simulink model "LotkaVolterra"  (R2024b)
settings: Solver=VariableStepAuto  StartTime=0.0  StopTime=10.0  RelTol=1e-3
settings Model: Creator=hp  LastModifiedBy=hp
settings DataIOCC: ReturnWorkspaceOutputs=off

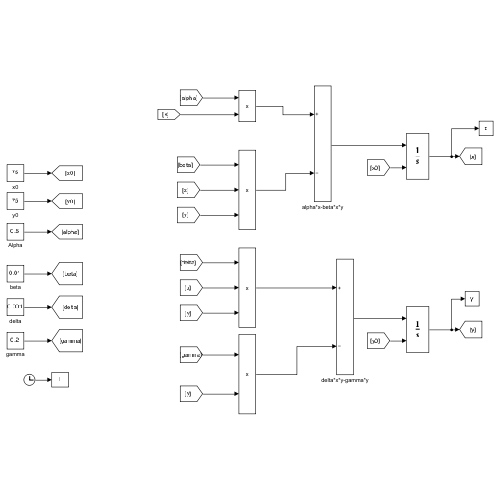
[thumbnail: Simulink's stored preview of the top-level diagram]
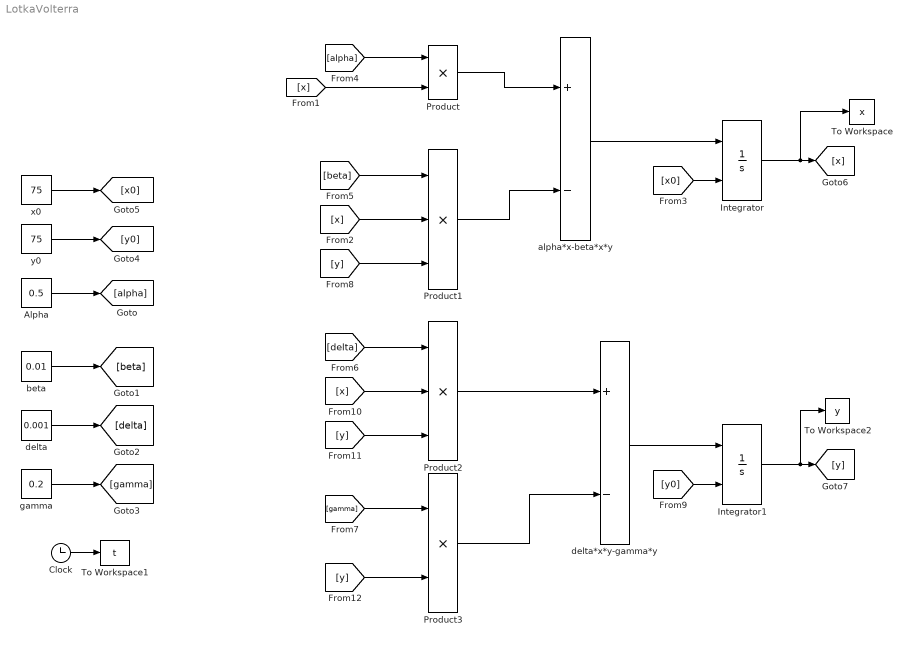
== system LotkaVolterra ==
  Alpha : Constant  Value=0.5
  Clock : Clock
  Integrator : Integrator  InitialConditionSource=external
  Integrator1 : Integrator  InitialConditionSource=external
  Product : Product
  Product1 : Product  Inputs=3
  Product2 : Product  Inputs=3
  Product3 : Product
  To Workspace : ToWorkspace  VariableName=x  SampleTime=-1
  To Workspace1 : ToWorkspace  VariableName=t  SampleTime=-1
  To Workspace2 : ToWorkspace  VariableName=y  SampleTime=-1
  alpha*x-beta*x*y : Sum  Inputs=+-
  beta : Constant  Value=0.01
  delta : Constant  Value=0.001
  delta*x*y-gamma*y : Sum  Inputs=+-
  gamma : Constant  Value=0.2
  x0 : Constant  Value=75
  y0 : Constant  Value=75
  wires:
  Alpha/1 -> [alpha]
  beta/1 -> [beta]
  delta/1 -> [delta]
  gamma/1 -> [gamma]
  y0/1 -> [y0]
  x0/1 -> [x0]
  [alpha] -> Product/1
  [x] -> Product/2
  [beta] -> Product1/1
  [x] -> Product1/2
  Product/1 -> alpha*x-beta*x*y/1
  Integrator/1 -> To Workspace/1, [x]
  [x0] -> Integrator/2
  alpha*x-beta*x*y/1 -> Integrator/1
  Product1/1 -> alpha*x-beta*x*y/2
  [y] -> Product1/3
  delta*x*y-gamma*y/1 -> Integrator1/1
  [y0] -> Integrator1/2
  Integrator1/1 -> To Workspace2/1, [y]
  Product2/1 -> delta*x*y-gamma*y/1
  [delta] -> Product2/1
  [x] -> Product2/2
  [y] -> Product2/3
  [gamma] -> Product3/1
  [y] -> Product3/2
  Product3/1 -> delta*x*y-gamma*y/2
  Clock/1 -> To Workspace1/1
